simulink model "psbctsat"  (Simulink 6.0)
settings: Solver=ode23tb  StartTime=0.0  StopTime=.2  MaxStep=100e-6  RelTol=1e-4
InitFcn:
  | powericon('psbinitsys',bdroot);
libraries: powerlib2 x12
settings Model: Creator=sybille  LastModifiedBy=batserve  ExtModeTrigMode=oneshot  ExtModeArmWhenConnect=off  ExtModeAutoUpdateStatusClock=off  ProdHWDeviceType=Specified
settings DataIOCC: LimitDataPoints=off  SignalLoggingName=sigsOut
settings OptimizationCC: BlockReduction=off  BooleanDataType=off
settings DebuggingCC: CheckExecutionContextPreStartOutputMsg=on  CheckExecutionContextRuntimeOutputMsg=on  SolverPrmCheckMsg=none
settings HardwareCC: ProdBitPerShort=32  ProdBitPerInt=16  ProdHWDeviceType=Specified  TargetUnknown=on

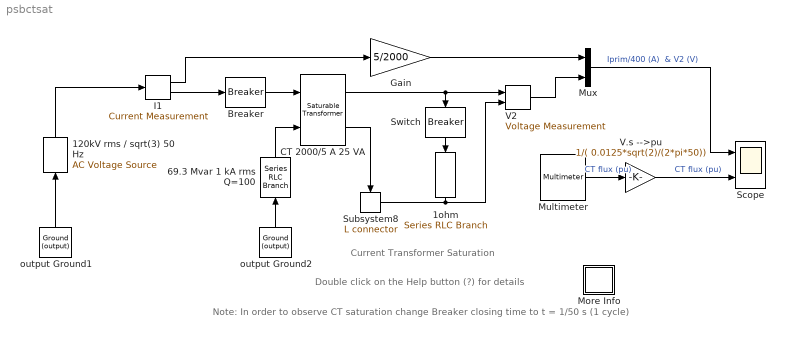
== system psbctsat ==
  note: Current Transformer Saturation
  note: Double click on the Help button (?) for details
  note: Note: In order to observe CT saturation
      | change Breaker closing time to t = 1/50 s (1 cycle)
  120kV rms / sqrt(3) 50 Hz : powerlib2/Electrical Sources/AC Voltage Source  Tag=PoWeRsYsTeMbLoCk  Description=source block  Orientation=up  A=120e3/sqrt(3)*sqrt(2)  P=0  F=50  stime=0  mesure=None  PSBOutputType=1
  1ohm : powerlib2/Elements/Series RLC Branch  Tag=PoWeRsYsTeMbLoCk  Orientation=down  a=1  b=0  c=inf  mesure=None  PSBOutputType=1
  69.3 Mvar 1 kA rms Q=100 : powerlib2/Elements/Series RLC Branch  Tag=PoWeRsYsTeMbLoCk  Orientation=up  a=69.3e3/1e3/100  b=69.3e3/1e3/(2*pi*50)  c=inf  mesure=None  PSBOutputType=1
  Breaker : powerlib2/Elements/Breaker  Tag=PoWeRsYsTeMbLoCk  a=0.01  c=0  rs=1e6  cs=inf  times=[ 1.25/50]  Ts=0  comext=off  mesure=None  PSBOutputType=1
  CT 2000/5 A 25 VA : powerlib2/Elements/Saturable Transformer  Tag=PoWeRsYsTeMbLoCk  a=[25 50]  b=[5*5/2000 0.001 0.04]  c=[5 0.001 0.04 ]  w3check=off  d=[5 0.001 0.04 ]  e=[0 0 ; 0.01 10 ; 1 10.5]  f=[100]  H=off  matfile='hysteresis'  Initialslope=+1  mesure=Flux and magnetization current ( Imag )  PSBOutputType=1111
  Gain : Gain  Gain=5/2000  SaturateOnIntegerOverflow=on
  I1 : powerlib2/Measurements/Current Measurement  Tag=PoWeRsYsTeMmEaSuReMeNt  PhasorSimulation=off  OutputType=Magnitude  PSBOutputType=01  PSBequivalent=0
  More Info : Subsystem
      mask Display: disp('?')
  Multimeter : powerlib2/Measurements/Multimeter  Tag=PoWeRsYsTeMmEaSuReMeNt  PhasorSimulation=off  OutputType=Magnitude  sel=2  L=2  Gain=1  yselected={'Flux: CT 2000//5 A 25 VA'};  PSBOutputType=1  PSBequivalent=0  AxesSetting=[0,0.1,-100,100]  Display=0  SavedBlockNames={}
  Mux : Mux  Inputs=2
  Scope : Scope  NumInputPorts=2
      settings: TimeRange=0.2  YMin=-4~-0.4  YMax=4~1
  Subsystem8 : powerlib2/Connectors/L connector  Tag=PoWeRsYsTeMbLoCk  Orientation=down
  Switch : powerlib2/Elements/Breaker  Tag=PoWeRsYsTeMbLoCk  Orientation=down  a=0.001  c=1  rs=1e6  cs=inf  times="[  99 ]"  Ts=0  comext=off  mesure=None  PSBOutputType=1
  V.s -->pu : Gain  Gain=1/( 0.0125*sqrt(2)/(2*pi*50))  SaturateOnIntegerOverflow=on
  V2 : powerlib2/Measurements/Voltage Measurement  Tag=PoWeRsYsTeMmEaSuReMeNt  PhasorSimulation=off  OutputType=Magnitude  PSBOutputType=0  PSBequivalent=0
  output Ground1 : powerlib2/Connectors/Ground (output)  Tag=PoWeRsYsTeMbLoCk  Orientation=up  PSBOutputType=1
  output Ground2 : powerlib2/Connectors/Ground (output)  Tag=PoWeRsYsTeMbLoCk  Orientation=up  PSBOutputType=1
  wires:
  output Ground1/1 -> 120kV rms / sqrt(3) 50 Hz/1
  120kV rms / sqrt(3) 50 Hz/1 -> I1/1
  I1/1 -> Gain/1
  Gain/1 -> Mux/1
  Mux/1 -> Scope/1  "Iprim/400 (A)  & V2 (V)"
  I1/2 -> Breaker/1
  Breaker/1 -> CT 2000/5 A 25 VA/1
  V2/1 -> Mux/2
  Multimeter/1 -> V.s -->pu/1  "CT flux (pu)"
  V.s -->pu/1 -> Scope/2  "CT flux (pu)"
  69.3 Mvar 1 kA rms Q=100/1 -> CT 2000/5 A 25 VA/2
  output Ground2/1 -> 69.3 Mvar 1 kA rms Q=100/1
  CT 2000/5 A 25 VA/2 -> Subsystem8/1
  CT 2000/5 A 25 VA/1 -> Switch/1, V2/1
  Switch/1 -> 1ohm/1
  1ohm/1 -> Subsystem8/Enable, V2/2

== system psbctsat/More Info ==
  note: 1. Normal operation
  note: In this test , the breaker  is closed at a peak of source voltage (t = 1.25 cycle). This switching produces no current asymmetry.
      | Start the simulation and observe the CT primary current and secondary voltage (first tace of Scope block).
      | As expected the the CT current and voltage are sinusoidal and the measurement error due to CT resistance and leakage
      | reactances is not significant. The flux contains a DC component but it stays lower than the 10 pu saturation value.
  note: Circuit Description
  note: This demonstration illustrates measurement distortion due to saturation of a current transformer (CT)
  note: A  current transformer (CT) is used to measure current in a shunt inductor connected on  a 120 kV network.
      | The CT is rated 2000 A / 5 A , 5 VA. The primary winding which consists of a single turn passing through the
      | CT toroidal core is connected in series with the shunt inductor rated 69.3 Mvar, 69.3 kV (120kV/sqrt(3)) , 1 kA rms.
      | The secondary  winding consisting of 1*2000/5 = 400 turns is short circuited through a 1 ohm load resistance.
      | A voltage sensor connected at the secondary reads a voltage which should be proportional to the primary current.
      | In steady state, the  current flowing in the secondary is 1000*5/2000 = 2.5 A   (2.5 Vrms or 3.54 Vpeak read by the
      | voltage mesurement block V2).
      |
      | Open the CT dialog box and observe how the CT parameters are specified.
      | The CT is assumed to saturate at 10 pu and a simple 2 segment saturation characteristic is used.
      |
      | The primary current reflected on the secondary and the voltage developped across the 1 ohm resistance are sent to
      | trace 1 of the Scope block. The CT flux , measured by the Multimeter block is converted in  pu and sent to trace 2.
      | (1 pu flux= 0.0125 V *sqrt(2)/ (2*pi*50)=5.63e-5 V.s)
      |
      | The switch connected in series with the CT secondary is normally closed.
      | This switch will be used later to illustrate overvoltages produced  when CT secondary is left open.
  note: Demonstration
  note: G. Sybille (Hydro-Quebec)
  note: 2. CT saturation due to current asymmetry
  note: Now, change the breaker closing time in order to close at a voltage zero crossing . Use t = 1/50 s.
      | This switching instant will now produce full current asymmetry in the shunt reactor. Restart the simulation.
      | Observe that for the first 3 cycles, the flux stays lower than the saturation knee point (10 pu).  The CT voltage output V2
      | then follows the primary current. However, after 3 cycles, the flux asymmetry produced by the primary current causes
      | CT saturation, thus producing large distortion of  CT secondary voltage.
  note: 3. Overvoltage due to CT secondary opening
  note: Reprogram the primary  breaker closing time at t = 1.25/50 s (no flux asymmetry) and change the secondary switch
      | opening time to t = 0.1 s. Restart the simulation and observe the large overvoltage produced  when the CT secondary is opened.
      | The flux has a square waveshape chopped at +10 and -10 pu. Large dphi/dt produced at flux inversion generates high
      | voltage spikes (250 V).
